simulink model "experiment"  (R2016a)
settings: Solver=VariableStepAuto  StartTime=0.0  StopTime=inf  RelTol=1e-3
undefined symbols (not defined in the file or in its folder): Ae, Be, Ce, d, De, l0, Tsample
libraries: etargetslib x2, dspnetwork x2, utility x1
settings Model: Creator=Florian  LastModifiedBy=Florian

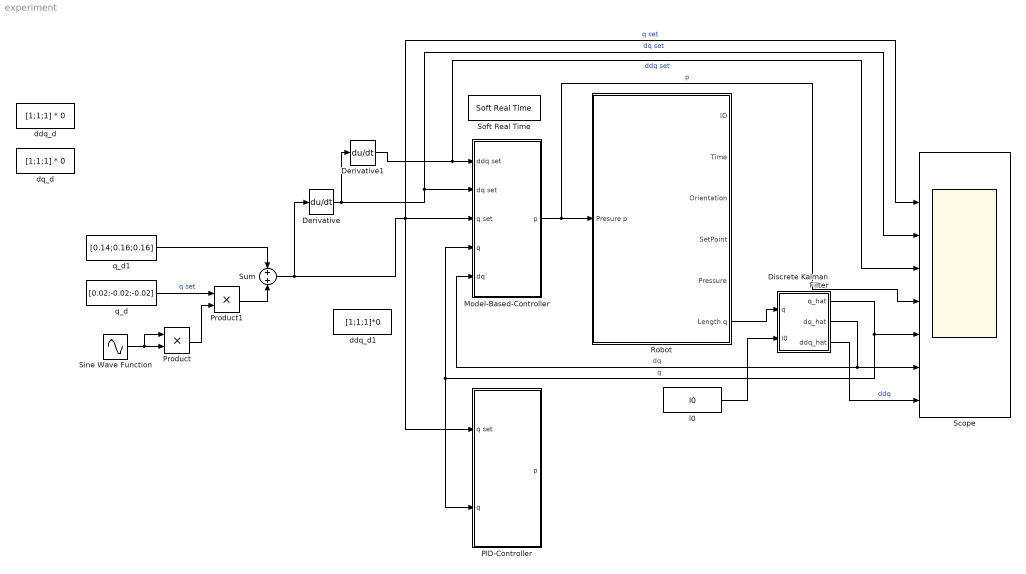
== system experiment ==
  Derivative : Derivative
  Derivative1 : Derivative
  Discrete Kalman Filter : MATLAB Function  TreatAsAtomicUnit=on  SystemSampleTime=Tsample
  Model-Based-Controller : Subsystem
  PID-Controller : Subsystem
  Product : Product
  Product1 : Product
  Robot : Subsystem
      mask Display: image('C:\Users\Florian\Documents\Uni\IDP\DVD\Pictures\contibot1seg.JPG');
  Scope : Scope  NumInputPorts=8
  Sine Wave Function : Sin  Frequency=3  SampleTime=0
  Soft Real Time : utility/Soft Real Time  x=1
  Sum : Sum
  ddq_d : Constant  Value=[1;1;1] * 0  SampleTime=0.01
  ddq_d1 : Constant  Value=[1;1;1]*0  SampleTime=0.01
  dq_d : Constant  Value=[1;1;1] * 0  SampleTime=0.01
  l0 : Constant  Value=l0  SampleTime=0.01
  q_d : Constant  Value=[0.02;-0.02;-0.02]  SampleTime=0.01
  q_d1 : Constant  Value=[0.14;0.16;0.16]  SampleTime=0.01
  wires:
  Robot/6(Length q) -> Discrete Kalman Filter/1(q)
  Discrete Kalman Filter/1(q_hat) -> Scope/6, PID-Controller/2(q), Model-Based-Controller/4(q)  "q"
  Discrete Kalman Filter/2(dq_hat) -> Model-Based-Controller/5(dq), Scope/7  "dq"
  Discrete Kalman Filter/3(ddq_hat) -> Scope/8  "ddq"
  Derivative1/1 -> Scope/4, Model-Based-Controller/1(ddq set)  "ddq set"
  Derivative/1 -> Derivative1/1, Scope/3, Model-Based-Controller/2(dq set)  "dq set"
  l0/1 -> Discrete Kalman Filter/2(l0)
  Sum/1 -> PID-Controller/1(q set), Scope/2, Model-Based-Controller/3(q set), Derivative/1  "q set"
  Model-Based-Controller/1(p) -> Robot/1(Presure p), Scope/5  "p"
  Sine Wave Function/1 -> Product/1, Product/2
  Product/1 -> Product1/2
  q_d/1 -> Product1/1  "q set"
  Product1/1 -> Sum/2
  q_d1/1 -> Sum/1

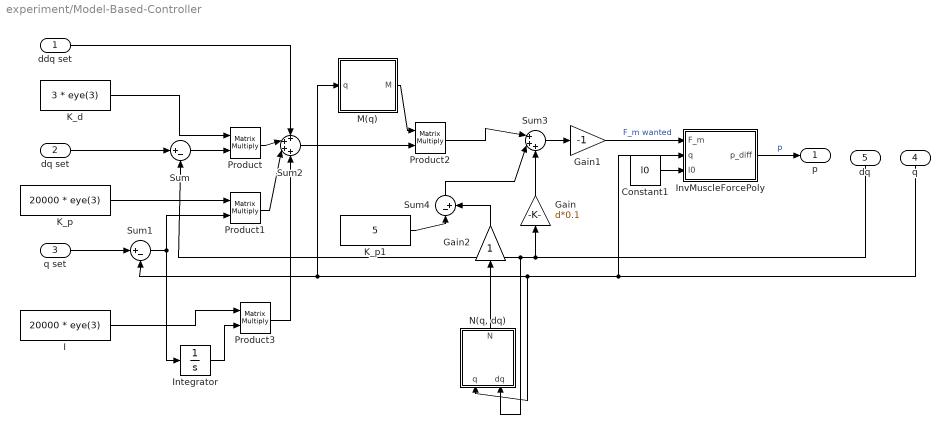
== system experiment/Model-Based-Controller ==
  ddq set : Inport
  dq set : Inport  Port=2
  q set : Inport  Port=3
  q : Inport  Port=4
  dq : Inport  Port=5
  Constant1 : Constant  Value=l0  SampleTime=0.01
  Gain : Gain  Gain=d*0.1
  Gain1 : Gain  Gain=-1
  Gain2 : Gain
  I : Constant  Value=20000 * eye(3)  SampleTime=0.01
  Integrator : Integrator  InitialCondition=[0;0;0]
  InvMuscleForcePoly : MATLAB Function  TreatAsAtomicUnit=on
  K_d : Constant  Value=3 * eye(3)  SampleTime=0.01
  K_p : Constant  Value=20000 * eye(3)  SampleTime=0.01
  K_p1 : Constant  Value=5  SampleTime=0.01
  M(q) : MATLAB Function  TreatAsAtomicUnit=on
  "N(q, dq)" : MATLAB Function  TreatAsAtomicUnit=on
  Product{,1..3} (4 alike) : Product  Multiplication=Matrix(*)
  Sum : Sum  Inputs=|+-
  Sum1 : Sum  Inputs=|+-
  Sum2 : Sum  Inputs=++++
  Sum3 : Sum  Inputs=|+++
  Sum4 : Sum  Inputs=|-+
  p : Outport
  wires:
  Sum/1 -> Product/2
  M(q)/1(M) -> Product2/1
  Sum2/1 -> Product2/2
  "N(q, dq)"/1(N) -> Gain2/1
  K_p/1 -> Product1/1
  Gain/1 -> Sum3/3
  Sum1/1 -> Product1/2, Integrator/1
  Product1/1 -> Sum2/3
  Product2/1 -> Sum3/1
  Product/1 -> Sum2/2
  Sum3/1 -> Gain1/1
  K_d/1 -> Product/1
  Constant1/1 -> InvMuscleForcePoly/3(l0)
  dq/1 -> Sum/2, "N(q, dq)"/2(dq), Gain/1
  q set/1 -> Sum1/1
  q/1 -> Sum1/2, M(q)/1(q), "N(q, dq)"/1(q), InvMuscleForcePoly/2(q)
  dq set/1 -> Sum/1
  ddq set/1 -> Sum2/1
  Gain2/1 -> Sum4/2
  Sum4/1 -> Sum3/2
  K_p1/1 -> Sum4/1
  Gain1/1 -> InvMuscleForcePoly/1(F_m)  "F_m wanted"
  InvMuscleForcePoly/1(p_diff) -> p/1  "p"
  Integrator/1 -> Product3/2
  I/1 -> Product3/1
  Product3/1 -> Sum2/4

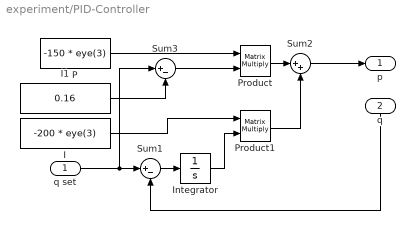
== system experiment/PID-Controller ==
  q set : Inport
  q : Inport  Port=2
  I : Constant  Value=-200 * eye(3)  SampleTime=0.01
  I1 : Constant  Value=0.16  SampleTime=0.01
  Integrator : Integrator  InitialCondition=[0;0;0]
  P : Constant  Value=-150 * eye(3)  SampleTime=0.01
  Product : Product  Multiplication=Matrix(*)
  Product1 : Product  Multiplication=Matrix(*)
  Sum1 : Sum  Inputs=|+-
  Sum2 : Sum  Inputs=|++
  Sum3 : Sum  Inputs=|+-
  p : Outport
  wires:
  I/1 -> Product1/1
  Product1/1 -> Sum2/2
  q set/1 -> Sum3/1, Sum1/1
  q/1 -> Sum1/2
  Product/1 -> Sum2/1
  Sum2/1 -> p/1
  Sum1/1 -> Integrator/1
  Integrator/1 -> Product1/2
  P/1 -> Product/1
  Sum3/1 -> Product/2
  I1/1 -> Sum3/2

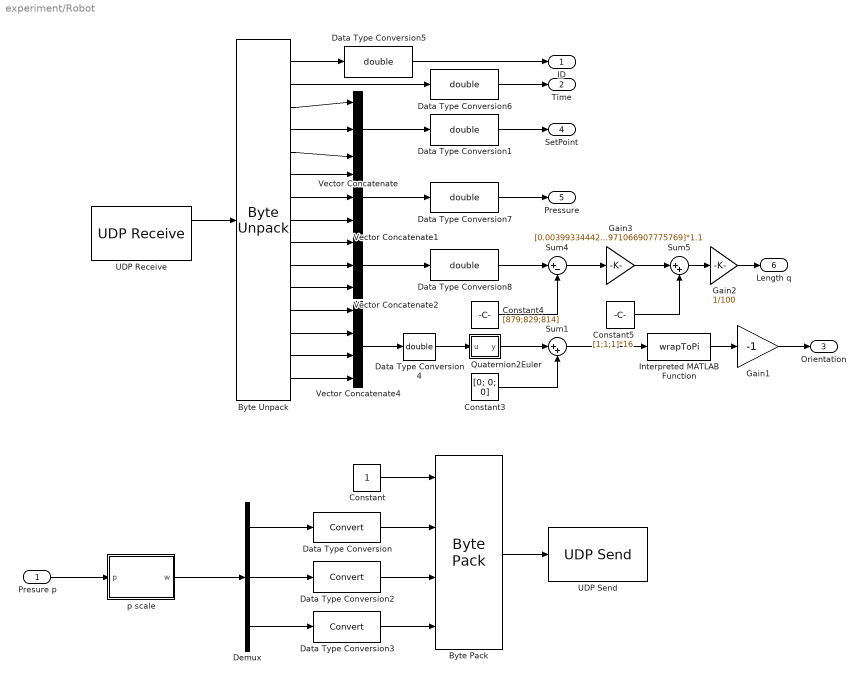
== system experiment/Robot ==
  Presure p : Inport
  Byte Pack : etargetslib/Byte Pack  datatypes={'uint32', 'uint32', 'uint32', 'uint32'}  byteAlign=1
  Byte Unpack : etargetslib/Byte Unpack  dimensions={[1],[1],[1],[1],[1],[1],[1],[1],[1],[1],[1],[1],[1],[1],[1]}  datatypes={'uint32', 'uint32', 'uint32', 'uint32', 'uint32', 'uint32', 'uint32', 'uint32', 'single', 'single', 'single', 'single', 'single', 'single', 'single'}  byteAlign=1
  Constant : Constant  OutDataTypeStr=uint32
  Constant3 : Constant  Value=[0; 0; 0]  OutDataTypeStr=uint32
  Constant4 : Constant  Value=[879;829;814]  OutDataTypeStr=uint32
  Constant5 : Constant  Value=[1;1;1]*16  OutDataTypeStr=uint32
  Data Type Conversion : DataTypeConversion
  Data Type Conversion{1,4..8} (6 alike) : DataTypeConversion  OutDataTypeStr=double
  Data Type Conversion2 : DataTypeConversion
  Data Type Conversion3 : DataTypeConversion
  Demux : Demux  Outputs=3
  Gain1 : Gain  Gain=-1
  Gain2 : Gain  Gain=1/100
  Gain3 : Gain  Gain=[0.00399334442595673876871880199667;0.0046332046332046332046332046332;0.00433996383363471971066907775769]*1.1
  Interpreted MATLAB Function : MATLABFcn  MATLABFcn=wrapToPi
  Quaternion2Euler : MATLAB Function  TreatAsAtomicUnit=on
  Sum1 : Sum  Inputs=|++
  Sum4 : Sum  Inputs=|+-
  Sum5 : Sum  Inputs=|++
  UDP Receive : dspnetwork/UDP Receive  localURL='0.0.0.0'  localPort=25000  remoteURL='0.0.0.0'  remotePort=-1  recvBufferSize=256  dims=15*4  signalDatatype=uint8  isVarSize=off  showBlockingTime=on  blockingTime=0  sampletime=Tsample  blockPlatform=HOST
  UDP Send : dspnetwork/UDP Send  remoteURL='127.0.0.1'  remotePort=12345  localURL='0.0.0.0'  localPortSource=Specify via dialog  localPort=25000  sampletime=-1  blockPlatform=HOST  separateLengthPort=0
  Vector Concatenate : Concatenate  NumInputs=3
  Vector Concatenate1 : Concatenate  NumInputs=3
  Vector Concatenate2 : Concatenate  NumInputs=3
  Vector Concatenate4 : Concatenate  NumInputs=4
  p scale : MATLAB Function  TreatAsAtomicUnit=on
  ID : Outport
  Time : Outport  Port=2
  Orientation : Outport  Port=3
  SetPoint : Outport  Port=4
  Pressure : Outport  Port=5
  Length q : Outport  Port=6
  wires:
  Gain1/1 -> Orientation/1
  Constant3/1 -> Sum1/2
  Sum1/1 -> Interpreted MATLAB Function/1
  Interpreted MATLAB Function/1 -> Gain1/1
  Byte Unpack/9 -> Vector Concatenate2/1
  Constant/1 -> Byte Pack/1
  Vector Concatenate/1 -> Data Type Conversion1/1
  Byte Unpack/6 -> Vector Concatenate1/1
  Byte Unpack/4 -> Vector Concatenate/2
  Byte Pack/1 -> UDP Send/1
  Byte Unpack/3 -> Vector Concatenate/1
  Byte Unpack/12 -> Vector Concatenate4/1
  Byte Unpack/5 -> Vector Concatenate/3
  Byte Unpack/13 -> Vector Concatenate4/2
  Byte Unpack/14 -> Vector Concatenate4/3
  UDP Receive/1 -> Byte Unpack/1
  Byte Unpack/10 -> Vector Concatenate2/2
  Byte Unpack/7 -> Vector Concatenate1/2
  Byte Unpack/8 -> Vector Concatenate1/3
  Byte Unpack/11 -> Vector Concatenate2/3
  Byte Unpack/15 -> Vector Concatenate4/4
  Quaternion2Euler/1(y) -> Sum1/1
  Vector Concatenate2/1 -> Data Type Conversion8/1
  Data Type Conversion1/1 -> SetPoint/1
  Byte Unpack/1 -> Data Type Conversion5/1
  Data Type Conversion5/1 -> ID/1
  Data Type Conversion6/1 -> Time/1
  Byte Unpack/2 -> Data Type Conversion6/1
  Vector Concatenate1/1 -> Data Type Conversion7/1
  Data Type Conversion7/1 -> Pressure/1
  Demux/1 -> Data Type Conversion/1
  Demux/2 -> Data Type Conversion2/1
  Presure p/1 -> p scale/1(p)
  Demux/3 -> Data Type Conversion3/1
  Vector Concatenate4/1 -> Data Type Conversion4/1
  Data Type Conversion4/1 -> Quaternion2Euler/1(u)
  Data Type Conversion/1 -> Byte Pack/2
  Data Type Conversion2/1 -> Byte Pack/3
  Data Type Conversion3/1 -> Byte Pack/4
  p scale/1(w) -> Demux/1
  Sum4/1 -> Gain3/1
  Gain3/1 -> Sum5/1
  Constant5/1 -> Sum5/2
  Sum5/1 -> Gain2/1
  Constant4/1 -> Sum4/2
  Data Type Conversion8/1 -> Sum4/1
  Gain2/1 -> Length q/1

== matlab function experiment/Model-Based-Controller/InvMuscleForcePoly ==
  data: F_m input; p_diff output; q input; l0 input
function p_diff = fcn(F_m, q, l0)
%#codegen

% coder.extrinsic('Pfunc');
% 
% p00 = 30.78; %1.85;
% p10 = 71.9;%91.44;
% p01 = -22.58;%-28.46;
% %p20 = -1.181;
% %p11 = -2.827;
% %p02 = 1.159;
% 
% h = (l0 - q)/l0 * 100;
% 
% p_diff = (F_m - p00 - p01*h) / p10;

%wurzel = sqrt((p10 + p11*h).^2 - 4 * p20 * (p00 + p01*h + p02*h.^2 - F_m));
%p_diff1 = (-p10-p11*h + wurzel)/(2*p20);
%p_diff2 = (-p10-p11*h - wurzel)/(2*p20);

%p_diff = max(p_diff1, p_diff2);

%p_diff = 0 * F_m;
%p_diff = Pfunc(F_m, q);

% p00 =       17.64;
% p10 =       82.44;
% p01 =      -40.53;
% p11 =      -2.827;
% p02 =       3.249;
% p12 =   -0.004285;
% p03 =    -0.07887;
% 
% h = (l0 - q)/l0 * 100;
% h = [1;1;1]*5;
% 
% 
% p_diff = (F_m - p00 - p01 * h - p02 * h.^2 - p03 * h.^3 + 17) ./ (p10 + p11 * h + p12 * h.^2);
% p_diff = F_m / 13;

p1 =   7.551e-05;
p2 =    -0.01115;
p3 =      0.6236;
p4 =      -9.759;

p_diff = p1*F_m.^3 + p2*F_m.^2 + p3*F_m + p4;

for i = 1:length(p_diff)
    if p_diff(i) < 0
        p_diff(i) = 0;
    elseif p_diff(i) > 6
        p_diff(i) = 6;
    end
end

== matlab function experiment/Robot/Quaternion2Euler ==
  data: u input; y output
function y = fcn(u)
%#codegen
u = u / 1000;
y = zeros(3,1);

y(1) = atan2(2*(u(1)*u(2)+u(3)*u(4)),1-2*(u(2)*u(2)+u(3)*u(3)));

if abs(2*(u(1)*u(3)-u(4)*u(2))) > 1
    y(2) = 0;
else
    y(2) = asin(2*(u(1)*u(3)-u(4)*u(2)));
end
y(3) = atan2(2*(u(1)*u(4)+u(2)*u(3)),1-2*(u(3)*u(3)+u(4)*u(4)));

== matlab function experiment/Model-Based-Controller/M(q) ==
  data: M output; q input
function M = fcn(q)
%#codegen

%coder.extrinsic('Mfunc');
if abs(q(1) - q(2)) < 0.0001 && abs(q(2) - q(3)) < 0.0001
    M = Mfunc(q - [0.0001; 0; 0]);
else
    M = Mfunc(q);
end
M = Mfunc2(q);

== matlab function experiment/Discrete Kalman Filter ==
  data: Ae parameter; Be parameter; Ce parameter; De parameter; q input; q_hat output; dq_hat output; ddq_hat output; l0 input
function [q_hat,dq_hat, ddq_hat] = fcn(Ae,Be,Ce,De,q, l0)
%#codegen
persistent x
if isempty(x)
   x = [l0, l0, l0; 0, 0, 0; 0, 0, 0];
end
 
q_hat = zeros(size(q));
dq_hat = q_hat;
ddq_hat = dq_hat;

for i = 1:length(q)
x_pred = Ae * x(:, i) + Be * q(i);
hat = Ce * x(:, i) + De * q(i);
x(:, i) = x_pred;

y_hat = hat(1);
x_hat = hat(2:4,1);

q_hat(i) = x_hat(1);
dq_hat(i) = x_hat(2);
ddq_hat(i) = x_hat(3);
end

== matlab function experiment/Robot/p scale ==
  data: p input; w output
function w = fcn(p)
%#codegen

w = (p/1.6 + 1.95) * 500;

== matlab function experiment/Model-Based-Controller/N(q, dq) ==
  data: N output; q input; dq input
function N = fcn(q, dq)
%#codegen

%coder.extrinsic('Nfunc');
if abs(q(1) - q(2)) < 0.0001 && abs(q(2) - q(3)) < 0.0001
   N = Nfunc2(q, dq);
else
   N = Nfunc2(q, dq);
end

%N = (q - 0.17) * 1900;
